simulink model "ChartWithPorts"  (Simulink 7.4)
settings: Solver=ode45  StartTime=0.0  StopTime=10.0  RelTol=1e-3
settings Model: Creator=dread  LastModifiedBy=dread

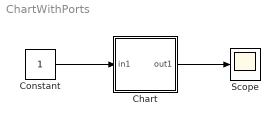
== system ChartWithPorts ==
  Chart : Stateflow chart
  Constant : Constant  OutDataType=fixdt(1, 16)  OutScaling=2^0
  Scope : Scope
  wires:
  Constant/1 -> Chart/1(in1)
  Chart/1(out1) -> Scope/1

== stateflow chart Chart ==
  state default
  (default) -> default : {out1 = in1;}
  data: in1 input double; out1 output double
